simulink model "Project1_SPXMMA001"  (R2021a)
settings: Solver=ode1  StartTime=0.0  StopTime=Inf  RelTol=1e-3
InitFcn:
  |  TOFF_InitialValue.PRE = 12000;
  | OFF_InitialValue.PRE = 12000;
  | TON_InitialValue.PRE = 2000;
  | ON_InitialValue.PRE = 2000;
  | T2OFF_InitialValue.PRE = 11000;
  | T2ON_InitialValue.PRE = 3000;
  | T3OFF_InitialValue.PRE = 5000;
undefined symbols (not defined in the file): BOOL, DINT, slplc
libraries: simulink x7
(part 1 of 13)
settings Model: EnablePacing=on  Creator=arnoldpretorius  LastModifiedBy=Franc
settings SolverCC: AlgebraicLoopSolver=TrustRegion
settings DebuggingCC: SFMachineParentedDataDiag=warning

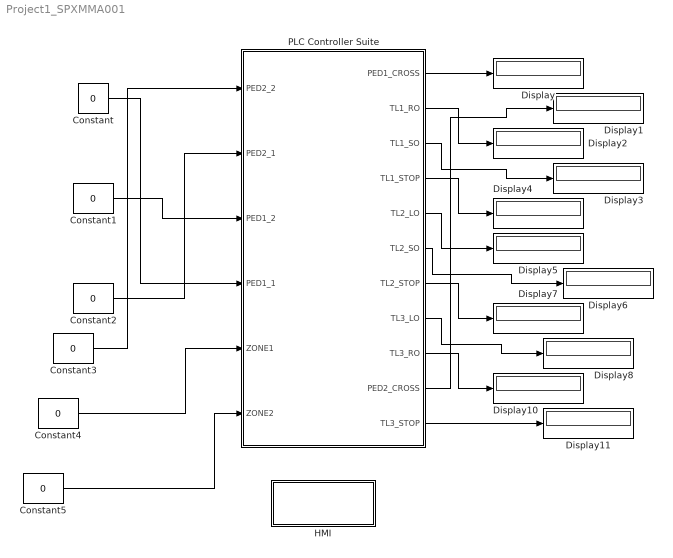
== system Project1_SPXMMA001 ==
  Constant{,1..5} (6 alike) : Constant  Value=0  OutDataTypeStr=boolean
  Display{,1..8,10..11} (11 alike) : Display
  HMI : Subsystem
  PLC Controller Suite : Subsystem  TreatAsAtomicUnit=on  mask{PLCBlockType=PLCController, PLCPOUType=PLC Controller}
      mask init:
      | slplc.callbacks.initController(gcb);
      settings: OpenFcn=slplc.callbacks.openPOUBlock(gcb);
      mask Help: web([docroot '/plccoder/ref/plccontrollersuite' '.html']);
      mask DialogControl PLCBlockTitle Prompt: PLC Controller Block
  wires:
  Constant/1 -> PLC Controller Suite/4(PED1_1)
  Constant1/1 -> PLC Controller Suite/3(PED1_2)
  Constant2/1 -> PLC Controller Suite/2(PED2_1)
  Constant3/1 -> PLC Controller Suite/1(PED2_2)
  PLC Controller Suite/1(PED1_CROSS) -> Display/1
  PLC Controller Suite/10(PED2_CROSS) -> Display1/1
  PLC Controller Suite/2(TL1_RO) -> Display2/1
  PLC Controller Suite/3(TL1_SO) -> Display3/1
  PLC Controller Suite/4(TL1_STOP) -> Display4/1
  PLC Controller Suite/5(TL2_LO) -> Display5/1
  PLC Controller Suite/6(TL2_SO) -> Display6/1
  PLC Controller Suite/7(TL2_STOP) -> Display7/1
  PLC Controller Suite/8(TL3_LO) -> Display8/1
  PLC Controller Suite/9(TL3_RO) -> Display10/1
  PLC Controller Suite/11(TL3_STOP) -> Display11/1
  Constant4/1 -> PLC Controller Suite/5(ZONE1)
  Constant5/1 -> PLC Controller Suite/6(ZONE2)

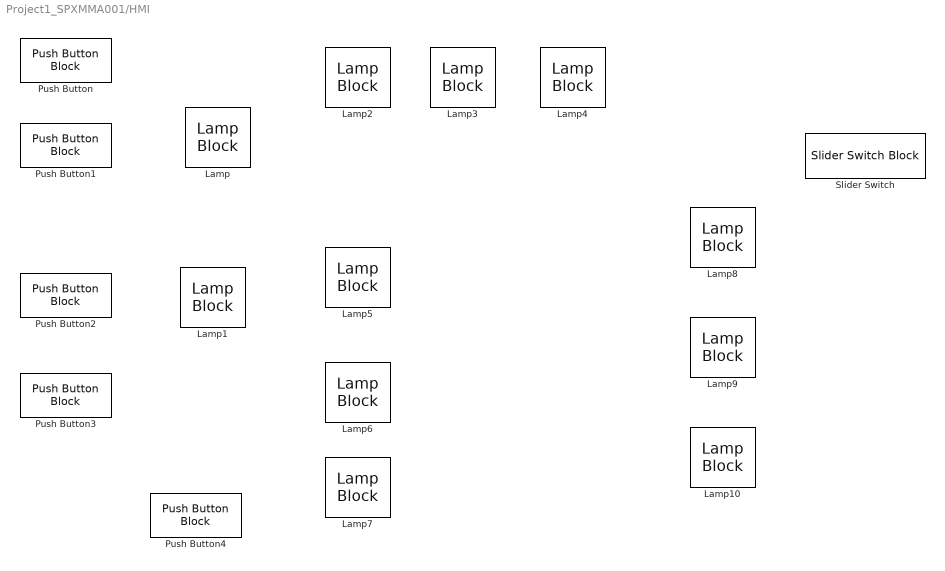
== system Project1_SPXMMA001/HMI ==
  Lamp{,1..10} (11 alike) : LampBlock
  Push Button : PushButtonBlock  ButtonText=PED1_1
  Push Button1 : PushButtonBlock  ButtonText=PED1_2
  Push Button2 : PushButtonBlock  ButtonText=PED2_1
  Push Button3 : PushButtonBlock  ButtonText=PED2_2
  Push Button4 : PushButtonBlock
  Slider Switch : SliderSwitchBlock  LabelPosition=Hide
      settings: Values={{'Off', 'On'}, [0 1]}

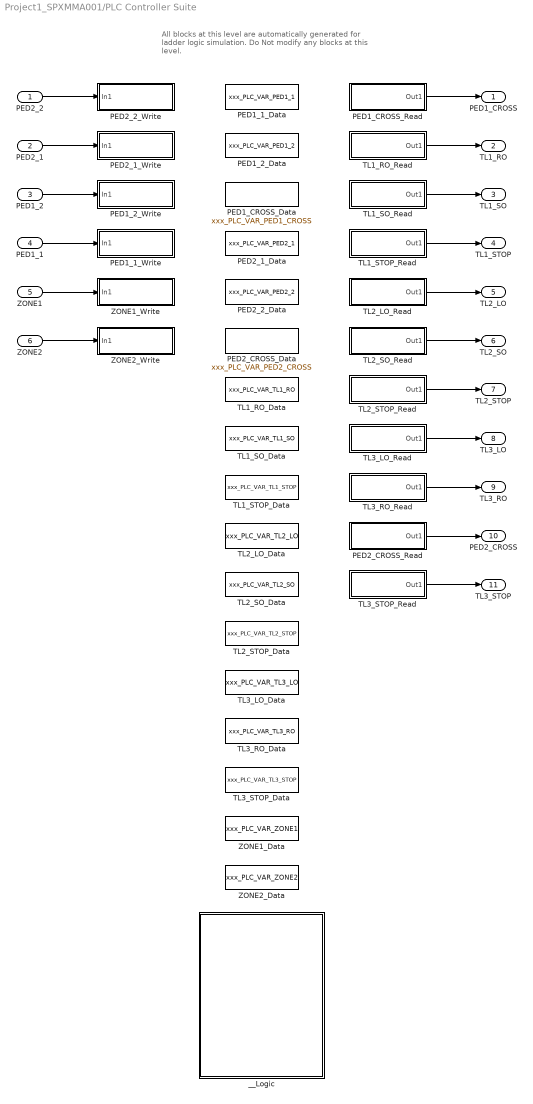
== system Project1_SPXMMA001/PLC Controller Suite ==
  note: All blocks at this level are automatically generated for ladder logic simulation.
      | Do Not modify any blocks at this level.
  PED2_2 : Inport  OutDataTypeStr=boolean
  PED2_1 : Inport  Port=2  OutDataTypeStr=boolean
  PED1_2 : Inport  Port=3  OutDataTypeStr=boolean
  PED1_1 : Inport  Port=4  OutDataTypeStr=boolean
  ZONE1 : Inport  Port=5  OutDataTypeStr=boolean
  ZONE2 : Inport  Port=6  OutDataTypeStr=boolean
  PED1_1_Data : DataStoreMemory  Tag=POUVariable  Priority=10  DataStoreName=xxx_PLC_VAR_PED1_1  ShowAdditionalParam=off  OutDataTypeStr=boolean  Dimensions=1
  PED1_1_Write : Subsystem  Priority=11  DisableCoverage=on  TreatAsAtomicUnit=on  mask{PLCOperandTag=PED1_1, PLCOperandExpression=xxx_PLC_VAR_PED1_1, PLCBlockType=VarWrite, PLCPOUType=VarWrite}
      mask prompts: PLCOperandTag "Operand Tag:"
      mask init:
      | slplc.callbacks.initInstruction(gcb);
      mask Help: web([docroot '/plccoder/ref/varwrite' '.html']);
      mask DialogControl PLCBlockTitle Prompt: Variable Write
      mask Display: disp(get_param(gcb, 'PLCOperandTag'));
  PED1_2_Data : DataStoreMemory  Tag=POUVariable  Priority=10  DataStoreName=xxx_PLC_VAR_PED1_2  ShowAdditionalParam=off  OutDataTypeStr=boolean  Dimensions=1
  PED1_2_Write : Subsystem  Priority=11  DisableCoverage=on  TreatAsAtomicUnit=on  mask{PLCOperandTag=PED1_2, PLCOperandExpression=xxx_PLC_VAR_PED1_2, PLCBlockType=VarWrite, PLCPOUType=VarWrite}
      mask prompts: PLCOperandTag "Operand Tag:"
      mask init:
      | slplc.callbacks.initInstruction(gcb);
      mask Help: web([docroot '/plccoder/ref/varwrite' '.html']);
      mask DialogControl PLCBlockTitle Prompt: Variable Write
      mask Display: disp(get_param(gcb, 'PLCOperandTag'));
  PED1_CROSS_Data : DataStoreMemory  Tag=POUVariable  Priority=10  DataStoreName=xxx_PLC_VAR_PED1_CROSS  ShowAdditionalParam=off  OutDataTypeStr=boolean  Dimensions=1
  PED1_CROSS_Read : Subsystem  Priority=13  DisableCoverage=on  TreatAsAtomicUnit=on  mask{PLCOperandTag=PED1_CROSS, PLCOperandExpression=xxx_PLC_VAR_PED1_CROSS, PLCBlockType=VarRead, PLCPOUType=VarRead}
      mask prompts: PLCOperandTag "Operand Tag"
      mask init:
      | block = gcb;
      | maskObj = Simulink.Mask.get(block);
      | maskObj.Display = sprintf('disp(''%s'');', PLCOperandTag);
      | slplc.callbacks.initInstruction(gcb);
      mask Help: web([docroot '/plccoder/ref/varread' '.html']);
      mask DialogControl PLCBlockTitle Prompt: Variable Read
      mask Display: disp('PED1_CROSS');
  PED2_1_Data : DataStoreMemory  Tag=POUVariable  Priority=10  DataStoreName=xxx_PLC_VAR_PED2_1  ShowAdditionalParam=off  OutDataTypeStr=boolean  Dimensions=1
  PED2_1_Write : Subsystem  Priority=11  DisableCoverage=on  TreatAsAtomicUnit=on  mask{PLCOperandTag=PED2_1, PLCOperandExpression=xxx_PLC_VAR_PED2_1, PLCBlockType=VarWrite, PLCPOUType=VarWrite}
      mask prompts: PLCOperandTag "Operand Tag:"
      mask init:
      | slplc.callbacks.initInstruction(gcb);
      mask Help: web([docroot '/plccoder/ref/varwrite' '.html']);
      mask DialogControl PLCBlockTitle Prompt: Variable Write
      mask Display: disp(get_param(gcb, 'PLCOperandTag'));
  PED2_2_Data : DataStoreMemory  Tag=POUVariable  Priority=10  DataStoreName=xxx_PLC_VAR_PED2_2  ShowAdditionalParam=off  OutDataTypeStr=boolean  Dimensions=1
  PED2_2_Write : Subsystem  Priority=11  DisableCoverage=on  TreatAsAtomicUnit=on  mask{PLCOperandTag=PED2_2, PLCOperandExpression=xxx_PLC_VAR_PED2_2, PLCBlockType=VarWrite, PLCPOUType=VarWrite}
      mask prompts: PLCOperandTag "Operand Tag:"
      mask init:
      | slplc.callbacks.initInstruction(gcb);
      mask Help: web([docroot '/plccoder/ref/varwrite' '.html']);
      mask DialogControl PLCBlockTitle Prompt: Variable Write
      mask Display: disp(get_param(gcb, 'PLCOperandTag'));
  PED2_CROSS_Data : DataStoreMemory  Tag=POUVariable  Priority=10  DataStoreName=xxx_PLC_VAR_PED2_CROSS  ShowAdditionalParam=off  OutDataTypeStr=boolean  Dimensions=1
  PED2_CROSS_Read : Subsystem  Priority=13  DisableCoverage=on  TreatAsAtomicUnit=on  mask{PLCOperandTag=PED2_CROSS, PLCOperandExpression=xxx_PLC_VAR_PED2_CROSS, PLCBlockType=VarRead, PLCPOUType=VarRead}
      mask prompts: PLCOperandTag "Operand Tag"
      mask init:
      | block = gcb;
      | maskObj = Simulink.Mask.get(block);
      | maskObj.Display = sprintf('disp(''%s'');', PLCOperandTag);
      | slplc.callbacks.initInstruction(gcb);
      mask Help: web([docroot '/plccoder/ref/varread' '.html']);
      mask DialogControl PLCBlockTitle Prompt: Variable Read
      mask Display: disp('PED2_CROSS');
  TL1_RO_Data : DataStoreMemory  Tag=POUVariable  Priority=10  DataStoreName=xxx_PLC_VAR_TL1_RO  ShowAdditionalParam=off  OutDataTypeStr=boolean  Dimensions=1
  TL1_RO_Read : Subsystem  Priority=13  DisableCoverage=on  TreatAsAtomicUnit=on  mask{PLCOperandTag=TL1_RO, PLCOperandExpression=xxx_PLC_VAR_TL1_RO, PLCBlockType=VarRead, PLCPOUType=VarRead}
      mask prompts: PLCOperandTag "Operand Tag"
      mask init:
      | block = gcb;
      | maskObj = Simulink.Mask.get(block);
      | maskObj.Display = sprintf('disp(''%s'');', PLCOperandTag);
      | slplc.callbacks.initInstruction(gcb);
      mask Help: web([docroot '/plccoder/ref/varread' '.html']);
      mask DialogControl PLCBlockTitle Prompt: Variable Read
      mask Display: disp('TL1_RO');
  TL1_SO_Data : DataStoreMemory  Tag=POUVariable  Priority=10  DataStoreName=xxx_PLC_VAR_TL1_SO  ShowAdditionalParam=off  OutDataTypeStr=boolean  Dimensions=1
  TL1_SO_Read : Subsystem  Priority=13  DisableCoverage=on  TreatAsAtomicUnit=on  mask{PLCOperandTag=TL1_SO, PLCOperandExpression=xxx_PLC_VAR_TL1_SO, PLCBlockType=VarRead, PLCPOUType=VarRead}
      mask prompts: PLCOperandTag "Operand Tag"
      mask init:
      | block = gcb;
      | maskObj = Simulink.Mask.get(block);
      | maskObj.Display = sprintf('disp(''%s'');', PLCOperandTag);
      | slplc.callbacks.initInstruction(gcb);
      mask Help: web([docroot '/plccoder/ref/varread' '.html']);
      mask DialogControl PLCBlockTitle Prompt: Variable Read
      mask Display: disp('TL1_SO');
  TL1_STOP_Data : DataStoreMemory  Tag=POUVariable  Priority=10  DataStoreName=xxx_PLC_VAR_TL1_STOP  ShowAdditionalParam=off  OutDataTypeStr=boolean  Dimensions=1
  TL1_STOP_Read : Subsystem  Priority=13  DisableCoverage=on  TreatAsAtomicUnit=on  mask{PLCOperandTag=TL1_STOP, PLCOperandExpression=xxx_PLC_VAR_TL1_STOP, PLCBlockType=VarRead, PLCPOUType=VarRead}
      mask prompts: PLCOperandTag "Operand Tag"
      mask init:
      | block = gcb;
      | maskObj = Simulink.Mask.get(block);
      | maskObj.Display = sprintf('disp(''%s'');', PLCOperandTag);
      | slplc.callbacks.initInstruction(gcb);
      mask Help: web([docroot '/plccoder/ref/varread' '.html']);
      mask DialogControl PLCBlockTitle Prompt: Variable Read
      mask Display: disp('TL1_STOP');
  TL2_LO_Data : DataStoreMemory  Tag=POUVariable  Priority=10  DataStoreName=xxx_PLC_VAR_TL2_LO  ShowAdditionalParam=off  OutDataTypeStr=boolean  Dimensions=1
  TL2_LO_Read : Subsystem  Priority=13  DisableCoverage=on  TreatAsAtomicUnit=on  mask{PLCOperandTag=TL2_LO, PLCOperandExpression=xxx_PLC_VAR_TL2_LO, PLCBlockType=VarRead, PLCPOUType=VarRead}
      mask prompts: PLCOperandTag "Operand Tag"
      mask init:
      | block = gcb;
      | maskObj = Simulink.Mask.get(block);
      | maskObj.Display = sprintf('disp(''%s'');', PLCOperandTag);
      | slplc.callbacks.initInstruction(gcb);
      mask Help: web([docroot '/plccoder/ref/varread' '.html']);
      mask DialogControl PLCBlockTitle Prompt: Variable Read
      mask Display: disp('TL2_LO');
  TL2_SO_Data : DataStoreMemory  Tag=POUVariable  Priority=10  DataStoreName=xxx_PLC_VAR_TL2_SO  ShowAdditionalParam=off  OutDataTypeStr=boolean  Dimensions=1
  TL2_SO_Read : Subsystem  Priority=13  DisableCoverage=on  TreatAsAtomicUnit=on  mask{PLCOperandTag=TL2_SO, PLCOperandExpression=xxx_PLC_VAR_TL2_SO, PLCBlockType=VarRead, PLCPOUType=VarRead}
      mask prompts: PLCOperandTag "Operand Tag"
      mask init:
      | block = gcb;
      | maskObj = Simulink.Mask.get(block);
      | maskObj.Display = sprintf('disp(''%s'');', PLCOperandTag);
      | slplc.callbacks.initInstruction(gcb);
      mask Help: web([docroot '/plccoder/ref/varread' '.html']);
      mask DialogControl PLCBlockTitle Prompt: Variable Read
      mask Display: disp('TL2_SO');
  TL2_STOP_Data : DataStoreMemory  Tag=POUVariable  Priority=10  DataStoreName=xxx_PLC_VAR_TL2_STOP  ShowAdditionalParam=off  OutDataTypeStr=boolean  Dimensions=1
  TL2_STOP_Read : Subsystem  Priority=13  DisableCoverage=on  TreatAsAtomicUnit=on  mask{PLCOperandTag=TL2_STOP, PLCOperandExpression=xxx_PLC_VAR_TL2_STOP, PLCBlockType=VarRead, PLCPOUType=VarRead}
      mask prompts: PLCOperandTag "Operand Tag"
      mask init:
      | block = gcb;
      | maskObj = Simulink.Mask.get(block);
      | maskObj.Display = sprintf('disp(''%s'');', PLCOperandTag);
      | slplc.callbacks.initInstruction(gcb);
      mask Help: web([docroot '/plccoder/ref/varread' '.html']);
      mask DialogControl PLCBlockTitle Prompt: Variable Read
      mask Display: disp('TL2_STOP');
  TL3_LO_Data : DataStoreMemory  Tag=POUVariable  Priority=10  DataStoreName=xxx_PLC_VAR_TL3_LO  ShowAdditionalParam=off  OutDataTypeStr=boolean  Dimensions=1
  TL3_LO_Read : Subsystem  Priority=13  DisableCoverage=on  TreatAsAtomicUnit=on  mask{PLCOperandTag=TL3_LO, PLCOperandExpression=xxx_PLC_VAR_TL3_LO, PLCBlockType=VarRead, PLCPOUType=VarRead}
      mask prompts: PLCOperandTag "Operand Tag"
      mask init:
      | block = gcb;
      | maskObj = Simulink.Mask.get(block);
      | maskObj.Display = sprintf('disp(''%s'');', PLCOperandTag);
      | slplc.callbacks.initInstruction(gcb);
      mask Help: web([docroot '/plccoder/ref/varread' '.html']);
      mask DialogControl PLCBlockTitle Prompt: Variable Read
      mask Display: disp('TL3_LO');
  TL3_RO_Data : DataStoreMemory  Tag=POUVariable  Priority=10  DataStoreName=xxx_PLC_VAR_TL3_RO  ShowAdditionalParam=off  OutDataTypeStr=boolean  Dimensions=1
  TL3_RO_Read : Subsystem  Priority=13  DisableCoverage=on  TreatAsAtomicUnit=on  mask{PLCOperandTag=TL3_RO, PLCOperandExpression=xxx_PLC_VAR_TL3_RO, PLCBlockType=VarRead, PLCPOUType=VarRead}
      mask prompts: PLCOperandTag "Operand Tag"
      mask init:
      | block = gcb;
      | maskObj = Simulink.Mask.get(block);
      | maskObj.Display = sprintf('disp(''%s'');', PLCOperandTag);
      | slplc.callbacks.initInstruction(gcb);
      mask Help: web([docroot '/plccoder/ref/varread' '.html']);
      mask DialogControl PLCBlockTitle Prompt: Variable Read
      mask Display: disp('TL3_RO');
  TL3_STOP_Data : DataStoreMemory  Tag=POUVariable  Priority=10  DataStoreName=xxx_PLC_VAR_TL3_STOP  ShowAdditionalParam=off  OutDataTypeStr=boolean  Dimensions=1
  TL3_STOP_Read : Subsystem  Priority=13  DisableCoverage=on  TreatAsAtomicUnit=on  mask{PLCOperandTag=TL3_STOP, PLCOperandExpression=xxx_PLC_VAR_TL3_STOP, PLCBlockType=VarRead, PLCPOUType=VarRead}
      mask prompts: PLCOperandTag "Operand Tag"
      mask init:
      | block = gcb;
      | maskObj = Simulink.Mask.get(block);
      | maskObj.Display = sprintf('disp(''%s'');', PLCOperandTag);
      | slplc.callbacks.initInstruction(gcb);
      mask Help: web([docroot '/plccoder/ref/varread' '.html']);
      mask DialogControl PLCBlockTitle Prompt: Variable Read
      mask Display: disp('TL3_STOP');
  ZONE1_Data : DataStoreMemory  Tag=POUVariable  Priority=10  DataStoreName=xxx_PLC_VAR_ZONE1  ShowAdditionalParam=off  OutDataTypeStr=boolean  Dimensions=1
  ZONE1_Write : Subsystem  Priority=11  DisableCoverage=on  TreatAsAtomicUnit=on  mask{PLCOperandTag=ZONE1, PLCOperandExpression=xxx_PLC_VAR_ZONE1, PLCBlockType=VarWrite, PLCPOUType=VarWrite}
      mask prompts: PLCOperandTag "Operand Tag:"
      mask init:
      | slplc.callbacks.initInstruction(gcb);
      mask Help: web([docroot '/plccoder/ref/varwrite' '.html']);
      mask DialogControl PLCBlockTitle Prompt: Variable Write
      mask Display: disp(get_param(gcb, 'PLCOperandTag'));
  ZONE2_Data : DataStoreMemory  Tag=POUVariable  Priority=10  DataStoreName=xxx_PLC_VAR_ZONE2  ShowAdditionalParam=off  OutDataTypeStr=boolean  Dimensions=1
  ZONE2_Write : Subsystem  Priority=11  DisableCoverage=on  TreatAsAtomicUnit=on  mask{PLCOperandTag=ZONE2, PLCOperandExpression=xxx_PLC_VAR_ZONE2, PLCBlockType=VarWrite, PLCPOUType=VarWrite}
      mask prompts: PLCOperandTag "Operand Tag:"
      mask init:
      | slplc.callbacks.initInstruction(gcb);
      mask Help: web([docroot '/plccoder/ref/varwrite' '.html']);
      mask DialogControl PLCBlockTitle Prompt: Variable Write
      mask Display: disp(get_param(gcb, 'PLCOperandTag'));
  __Logic : Subsystem  Priority=12  TreatAsAtomicUnit=on
  PED1_CROSS : Outport
  TL1_RO : Outport  Port=2
  TL1_SO : Outport  Port=3
  TL1_STOP : Outport  Port=4
  TL2_LO : Outport  Port=5
  TL2_SO : Outport  Port=6
  TL2_STOP : Outport  Port=7
  TL3_LO : Outport  Port=8
  TL3_RO : Outport  Port=9
  PED2_CROSS : Outport  Port=10
  TL3_STOP : Outport  Port=11
  wires:
  PED1_1/1 -> PED1_1_Write/1(In1)
  PED1_2/1 -> PED1_2_Write/1(In1)
  PED2_1/1 -> PED2_1_Write/1(In1)
  PED2_2/1 -> PED2_2_Write/1(In1)
  PED1_CROSS_Read/1(Out1) -> PED1_CROSS/1
  PED2_CROSS_Read/1(Out1) -> PED2_CROSS/1
  TL1_RO_Read/1(Out1) -> TL1_RO/1
  TL1_SO_Read/1(Out1) -> TL1_SO/1
  TL1_STOP_Read/1(Out1) -> TL1_STOP/1
  TL2_LO_Read/1(Out1) -> TL2_LO/1
  TL2_SO_Read/1(Out1) -> TL2_SO/1
  TL2_STOP_Read/1(Out1) -> TL2_STOP/1
  TL3_LO_Read/1(Out1) -> TL3_LO/1
  TL3_RO_Read/1(Out1) -> TL3_RO/1
  TL3_STOP_Read/1(Out1) -> TL3_STOP/1
  ZONE1/1 -> ZONE1_Write/1(In1)
  ZONE2/1 -> ZONE2_Write/1(In1)

== system Project1_SPXMMA001/PLC Controller Suite/PED1_1_Write ==
  In1 : Inport
  __CoreVarWrite : Subsystem  Tag=CoreVarWriteBlock  DisableCoverage=on  TreatAsAtomicUnit=on  mask{PLCBlockType=CoreVarWrite}
      mask init:
      | slplc.callbacks.initCoreVariable(gcb, 'write');
      mask DialogControl PLCBlockTitle Prompt: Core Variable Write
  wires:
  In1/1 -> __CoreVarWrite/1(u)

== system Project1_SPXMMA001/PLC Controller Suite/PED1_2_Write ==
  In1 : Inport
  __CoreVarWrite : Subsystem  Tag=CoreVarWriteBlock  DisableCoverage=on  TreatAsAtomicUnit=on  mask{PLCBlockType=CoreVarWrite}
      mask init:
      | slplc.callbacks.initCoreVariable(gcb, 'write');
      mask DialogControl PLCBlockTitle Prompt: Core Variable Write
  wires:
  In1/1 -> __CoreVarWrite/1(u)

== system Project1_SPXMMA001/PLC Controller Suite/PED1_CROSS_Read ==
  __CoreVarRead : Subsystem  Tag=CoreVarReadBlock  DisableCoverage=on  TreatAsAtomicUnit=on  mask{PLCBlockType=CoreVarRead}
      mask init:
      | slplc.callbacks.initCoreVariable(gcb, 'read');
      mask DialogControl PLCBlockTitle Prompt: Core Variable Read
  Out1 : Outport  VectorParamsAs1DForOutWhenUnconnected=off
  wires:
  __CoreVarRead/1(y) -> Out1/1

== system Project1_SPXMMA001/PLC Controller Suite/PED2_1_Write ==
  In1 : Inport
  __CoreVarWrite : Subsystem  Tag=CoreVarWriteBlock  DisableCoverage=on  TreatAsAtomicUnit=on  mask{PLCBlockType=CoreVarWrite}
      mask init:
      | slplc.callbacks.initCoreVariable(gcb, 'write');
      mask DialogControl PLCBlockTitle Prompt: Core Variable Write
  wires:
  In1/1 -> __CoreVarWrite/1(u)

== system Project1_SPXMMA001/PLC Controller Suite/PED2_2_Write ==
  In1 : Inport
  __CoreVarWrite : Subsystem  Tag=CoreVarWriteBlock  DisableCoverage=on  TreatAsAtomicUnit=on  mask{PLCBlockType=CoreVarWrite}
      mask init:
      | slplc.callbacks.initCoreVariable(gcb, 'write');
      mask DialogControl PLCBlockTitle Prompt: Core Variable Write
  wires:
  In1/1 -> __CoreVarWrite/1(u)

== system Project1_SPXMMA001/PLC Controller Suite/PED2_CROSS_Read ==
  __CoreVarRead : Subsystem  Tag=CoreVarReadBlock  DisableCoverage=on  TreatAsAtomicUnit=on  mask{PLCBlockType=CoreVarRead}
      mask init:
      | slplc.callbacks.initCoreVariable(gcb, 'read');
      mask DialogControl PLCBlockTitle Prompt: Core Variable Read
  Out1 : Outport  VectorParamsAs1DForOutWhenUnconnected=off
  wires:
  __CoreVarRead/1(y) -> Out1/1

== system Project1_SPXMMA001/PLC Controller Suite/TL1_RO_Read ==
  __CoreVarRead : Subsystem  Tag=CoreVarReadBlock  DisableCoverage=on  TreatAsAtomicUnit=on  mask{PLCBlockType=CoreVarRead}
      mask init:
      | slplc.callbacks.initCoreVariable(gcb, 'read');
      mask DialogControl PLCBlockTitle Prompt: Core Variable Read
  Out1 : Outport  VectorParamsAs1DForOutWhenUnconnected=off
  wires:
  __CoreVarRead/1(y) -> Out1/1

== system Project1_SPXMMA001/PLC Controller Suite/TL1_SO_Read ==
  __CoreVarRead : Subsystem  Tag=CoreVarReadBlock  DisableCoverage=on  TreatAsAtomicUnit=on  mask{PLCBlockType=CoreVarRead}
      mask init:
      | slplc.callbacks.initCoreVariable(gcb, 'read');
      mask DialogControl PLCBlockTitle Prompt: Core Variable Read
  Out1 : Outport  VectorParamsAs1DForOutWhenUnconnected=off
  wires:
  __CoreVarRead/1(y) -> Out1/1

== system Project1_SPXMMA001/PLC Controller Suite/TL1_STOP_Read ==
  __CoreVarRead : Subsystem  Tag=CoreVarReadBlock  DisableCoverage=on  TreatAsAtomicUnit=on  mask{PLCBlockType=CoreVarRead}
      mask init:
      | slplc.callbacks.initCoreVariable(gcb, 'read');
      mask DialogControl PLCBlockTitle Prompt: Core Variable Read
  Out1 : Outport  VectorParamsAs1DForOutWhenUnconnected=off
  wires:
  __CoreVarRead/1(y) -> Out1/1

== system Project1_SPXMMA001/PLC Controller Suite/TL2_LO_Read ==
  __CoreVarRead : Subsystem  Tag=CoreVarReadBlock  DisableCoverage=on  TreatAsAtomicUnit=on  mask{PLCBlockType=CoreVarRead}
      mask init:
      | slplc.callbacks.initCoreVariable(gcb, 'read');
      mask DialogControl PLCBlockTitle Prompt: Core Variable Read
  Out1 : Outport  VectorParamsAs1DForOutWhenUnconnected=off
  wires:
  __CoreVarRead/1(y) -> Out1/1

== system Project1_SPXMMA001/PLC Controller Suite/TL2_SO_Read ==
  __CoreVarRead : Subsystem  Tag=CoreVarReadBlock  DisableCoverage=on  TreatAsAtomicUnit=on  mask{PLCBlockType=CoreVarRead}
      mask init:
      | slplc.callbacks.initCoreVariable(gcb, 'read');
      mask DialogControl PLCBlockTitle Prompt: Core Variable Read
  Out1 : Outport  VectorParamsAs1DForOutWhenUnconnected=off
  wires:
  __CoreVarRead/1(y) -> Out1/1

== system Project1_SPXMMA001/PLC Controller Suite/TL2_STOP_Read ==
  __CoreVarRead : Subsystem  Tag=CoreVarReadBlock  DisableCoverage=on  TreatAsAtomicUnit=on  mask{PLCBlockType=CoreVarRead}
      mask init:
      | slplc.callbacks.initCoreVariable(gcb, 'read');
      mask DialogControl PLCBlockTitle Prompt: Core Variable Read
  Out1 : Outport  VectorParamsAs1DForOutWhenUnconnected=off
  wires:
  __CoreVarRead/1(y) -> Out1/1

== system Project1_SPXMMA001/PLC Controller Suite/TL3_LO_Read ==
  __CoreVarRead : Subsystem  Tag=CoreVarReadBlock  DisableCoverage=on  TreatAsAtomicUnit=on  mask{PLCBlockType=CoreVarRead}
      mask init:
      | slplc.callbacks.initCoreVariable(gcb, 'read');
      mask DialogControl PLCBlockTitle Prompt: Core Variable Read
  Out1 : Outport  VectorParamsAs1DForOutWhenUnconnected=off
  wires:
  __CoreVarRead/1(y) -> Out1/1

== system Project1_SPXMMA001/PLC Controller Suite/TL3_RO_Read ==
  __CoreVarRead : Subsystem  Tag=CoreVarReadBlock  DisableCoverage=on  TreatAsAtomicUnit=on  mask{PLCBlockType=CoreVarRead}
      mask init:
      | slplc.callbacks.initCoreVariable(gcb, 'read');
      mask DialogControl PLCBlockTitle Prompt: Core Variable Read
  Out1 : Outport  VectorParamsAs1DForOutWhenUnconnected=off
  wires:
  __CoreVarRead/1(y) -> Out1/1

== system Project1_SPXMMA001/PLC Controller Suite/TL3_STOP_Read ==
  __CoreVarRead : Subsystem  Tag=CoreVarReadBlock  DisableCoverage=on  TreatAsAtomicUnit=on  mask{PLCBlockType=CoreVarRead}
      mask init:
      | slplc.callbacks.initCoreVariable(gcb, 'read');
      mask DialogControl PLCBlockTitle Prompt: Core Variable Read
  Out1 : Outport  VectorParamsAs1DForOutWhenUnconnected=off
  wires:
  __CoreVarRead/1(y) -> Out1/1

== system Project1_SPXMMA001/PLC Controller Suite/ZONE1_Write ==
  In1 : Inport
  __CoreVarWrite : Subsystem  Tag=CoreVarWriteBlock  DisableCoverage=on  TreatAsAtomicUnit=on  mask{PLCBlockType=CoreVarWrite}
      mask init:
      | slplc.callbacks.initCoreVariable(gcb, 'write');
      mask DialogControl PLCBlockTitle Prompt: Core Variable Write
  wires:
  In1/1 -> __CoreVarWrite/1(u)

== system Project1_SPXMMA001/PLC Controller Suite/ZONE2_Write ==
  In1 : Inport
  __CoreVarWrite : Subsystem  Tag=CoreVarWriteBlock  DisableCoverage=on  TreatAsAtomicUnit=on  mask{PLCBlockType=CoreVarWrite}
      mask init:
      | slplc.callbacks.initCoreVariable(gcb, 'write');
      mask DialogControl PLCBlockTitle Prompt: Core Variable Write
  wires:
  In1/1 -> __CoreVarWrite/1(u)

== system Project1_SPXMMA001/PLC Controller Suite/__Logic ==
  Controller Tags : Subsystem  Tag=ControllerVariableSS  DisableCoverage=on  TreatAsAtomicUnit=on  mask{PLCVarPED2_2Name=PED2_2, PLCVarPED2_2Address=<empty>, PLCVarPED2_2Mapping=Input Symbol, PLCVarPED2_2PortIndex=1, PLCVarPED2_2DataType=boolean, PLCVarPED2_2Size=1, PLCVarPED2_2InitialValue=0, PLCVarPED2_2ToDelete=off, PLCVarPED2_1Name=PED2_1, PLCVarPED2_1Address=<empty>, PLCVarPED2_1Mapping=Input Symbol, PLCVarPED2_1PortIndex=2, PLCVarPED2_1DataType=boolean, PLCVarPED2_1Size=1, PLCVarPED2_1InitialValue=0, PLCVarPED2_1ToDelete=off, PLCVarPED1_2Name=PED1_2, PLCVarPED1_2Address=<empty>, PLCVarPED1_2Mapping=Input Symbol, PLCVarPED1_2PortIndex=3, PLCVarPED1_2DataType=boolean, PLCVarPED1_2Size=1, PLCVarPED1_2InitialValue=0, PLCVarPED1_2ToDelete=off, PLCVarPED1_1Name=PED1_1, PLCVarPED1_1Address=<empty>, PLCVarPED1_1Mapping=Input Symbol, PLCVarPED1_1PortIndex=4, PLCVarPED1_1DataType=boolean, PLCVarPED1_1Size=1, PLCVarPED1_1InitialValue=0, PLCVarPED1_1ToDelete=off, PLCVarZONE1Name=ZONE1, PLCVarZONE1Address=<empty>, PLCVarZONE1Mapping=Input Symbol, PLCVarZONE1PortIndex=5, PLCVarZONE1DataType=boolean, PLCVarZONE1Size=1, PLCVarZONE1InitialValue=0, PLCVarZONE1ToDelete=off, PLCVarZONE2Name=ZONE2, PLCVarZONE2Address=<empty>, PLCVarZONE2Mapping=Input Symbol, PLCVarZONE2PortIndex=6, PLCVarZONE2DataType=boolean, PLCVarZONE2Size=1, PLCVarZONE2InitialValue=0, PLCVarZONE2ToDelete=off, PLCVarPED1_CROSSName=PED1_CROSS, PLCVarPED1_CROSSAddress=<empty>, PLCVarPED1_CROSSMapping=Output Symbol, PLCVarPED1_CROSSPortIndex=1, PLCVarPED1_CROSSDataType=boolean, PLCVarPED1_CROSSSize=1, PLCVarPED1_CROSSInitialValue=0, PLCVarPED1_CROSSToDelete=off, PLCVarTL1_ROName=TL1_RO, PLCVarTL1_ROAddress=<empty>, PLCVarTL1_ROMapping=Output Symbol, PLCVarTL1_ROPortIndex=2, PLCVarTL1_RODataType=boolean, PLCVarTL1_ROSize=1, PLCVarTL1_ROInitialValue=0, PLCVarTL1_ROToDelete=off, PLCVarTL1_SOName=TL1_SO, PLCVarTL1_SOAddress=<empty>, PLCVarTL1_SOMapping=Output Symbol, PLCVarTL1_SOPortIndex=3, PLCVarTL1_SODataType=boolean, PLCVarTL1_SOSize=1, PLCVarTL1_SOInitialValue=0, PLCVarTL1_SOToDelete=off, PLCVarTL1_STOPName=TL1_STOP, PLCVarTL1_STOPAddress=<empty>, PLCVarTL1_STOPMapping=Output Symbol, PLCVarTL1_STOPPortIndex=4, PLCVarTL1_STOPDataType=boolean, PLCVarTL1_STOPSize=1, PLCVarTL1_STOPInitialValue=0, PLCVarTL1_STOPToDelete=off, PLCVarTL2_LOName=TL2_LO, PLCVarTL2_LOAddress=<empty>, PLCVarTL2_LOMapping=Output Symbol, PLCVarTL2_LOPortIndex=5, PLCVarTL2_LODataType=boolean, PLCVarTL2_LOSize=1, PLCVarTL2_LOInitialValue=0, PLCVarTL2_LOToDelete=off, PLCVarTL2_SOName=TL2_SO, PLCVarTL2_SOAddress=<empty>, PLCVarTL2_SOMapping=Output Symbol, PLCVarTL2_SOPortIndex=6, PLCVarTL2_SODataType=boolean, PLCVarTL2_SOSize=1, PLCVarTL2_SOInitialValue=0, PLCVarTL2_SOToDelete=off, PLCVarTL2_STOPName=TL2_STOP, PLCVarTL2_STOPAddress=<empty>, PLCVarTL2_STOPMapping=Output Symbol, PLCVarTL2_STOPPortIndex=7, PLCVarTL2_STOPDataType=boolean, PLCVarTL2_STOPSize=1, PLCVarTL2_STOPInitialValue=0, PLCVarTL2_STOPToDelete=off, PLCVarTL3_LOName=TL3_LO, PLCVarTL3_LOAddress=<empty>, PLCVarTL3_LOMapping=Output Symbol, PLCVarTL3_LOPortIndex=8, PLCVarTL3_LODataType=boolean, PLCVarTL3_LOSize=1, PLCVarTL3_LOInitialValue=0, PLCVarTL3_LOToDelete=off, PLCVarTL3_ROName=TL3_RO, PLCVarTL3_ROAddress=<empty>, PLCVarTL3_ROMapping=Output Symbol, PLCVarTL3_ROPortIndex=9, PLCVarTL3_RODataType=boolean, PLCVarTL3_ROSize=1, PLCVarTL3_ROInitialValue=0, PLCVarTL3_ROToDelete=off, PLCVarPED2_CROSSName=PED2_CROSS, PLCVarPED2_CROSSAddress=<empty>, PLCVarPED2_CROSSMapping=Output Symbol, PLCVarPED2_CROSSPortIndex=10, PLCVarPED2_CROSSDataType=boolean, PLCVarPED2_CROSSSize=1, PLCVarPED2_CROSSInitialValue=0, PLCVarPED2_CROSSToDelete=off, PLCVarTL3_STOPName=TL3_STOP, PLCVarTL3_STOPAddress=<empty>, PLCVarTL3_STOPMapping=Output Symbol, PLCVarTL3_STOPPortIndex=11, PLCVarTL3_STOPDataType=boolean, PLCVarTL3_STOPSize=1, PLCVarTL3_STOPInitialValue=0, PLCVarTL3_STOPToDelete=off}
      mask init:
      | slplc.callbacks.initControllerVarSS(gcb);
      settings: OpenFcn=slplc.callbacks.openControllerVariableSS(gcb);
      mask Help: web([docroot '/plccoder/ref/controllertags' '.html']);
      mask TypeOptions PLCVarPED2_2Mapping: Global Variable | Input Symbol | Output Symbol
      mask Callback PLCVarPED2_2Mapping: slplc.callbacks.updateControllerVarSS(gcb);
      mask TypeOptions PLCVarPED2_2PortIndex: 1 | 2 | 3 | 4 | 5 | 6 | 7 | 8 | 9 | 10 | 11 | 12 | 13 | 14 | 15 | 16 | 17
      mask TypeOptions PLCVarPED2_1Mapping: Global Variable | Input Symbol | Output Symbol
      mask Callback PLCVarPED2_1Mapping: slplc.callbacks.updateControllerVarSS(gcb);
      mask TypeOptions PLCVarPED2_1PortIndex: 1 | 2 | 3 | 4 | 5 | 6 | 7 | 8 | 9 | 10 | 11 | 12 | 13 | 14 | 15 | 16 | 17
      mask TypeOptions PLCVarPED1_2Mapping: Global Variable | Input Symbol | Output Symbol
      mask Callback PLCVarPED1_2Mapping: slplc.callbacks.updateControllerVarSS(gcb);
      mask TypeOptions PLCVarPED1_2PortIndex: 1 | 2 | 3 | 4 | 5 | 6 | 7 | 8 | 9 | 10 | 11 | 12 | 13 | 14 | 15 | 16 | 17
      mask TypeOptions PLCVarPED1_1Mapping: Global Variable | Input Symbol | Output Symbol
      mask Callback PLCVarPED1_1Mapping: slplc.callbacks.updateControllerVarSS(gcb);
      mask TypeOptions PLCVarPED1_1PortIndex: 1 | 2 | 3 | 4 | 5 | 6 | 7 | 8 | 9 | 10 | 11 | 12 | 13 | 14 | 15 | 16 | 17
      mask TypeOptions PLCVarZONE1Mapping: Global Variable | Input Symbol | Output Symbol
      mask Callback PLCVarZONE1Mapping: slplc.callbacks.updateControllerVarSS(gcb);
      mask TypeOptions PLCVarZONE1PortIndex: 1 | 2 | 3 | 4 | 5 | 6 | 7 | 8 | 9 | 10 | 11 | 12 | 13 | 14 | 15 | 16 | 17
      mask TypeOptions PLCVarZONE2Mapping: Global Variable | Input Symbol | Output Symbol
      mask Callback PLCVarZONE2Mapping: slplc.callbacks.updateControllerVarSS(gcb);
      mask TypeOptions PLCVarZONE2PortIndex: 1 | 2 | 3 | 4 | 5 | 6 | 7 | 8 | 9 | 10 | 11 | 12 | 13 | 14 | 15 | 16 | 17
      mask TypeOptions PLCVarPED1_CROSSMapping: Global Variable | Input Symbol | Output Symbol
      mask Callback PLCVarPED1_CROSSMapping: slplc.callbacks.updateControllerVarSS(gcb);
      mask TypeOptions PLCVarPED1_CROSSPortIndex: 1 | 2 | 3 | 4 | 5 | 6 | 7 | 8 | 9 | 10 | 11 | 12 | 13 | 14 | 15 | 16 | 17
      mask TypeOptions PLCVarTL1_ROMapping: Global Variable | Input Symbol | Output Symbol
      mask Callback PLCVarTL1_ROMapping: slplc.callbacks.updateControllerVarSS(gcb);
      mask TypeOptions PLCVarTL1_ROPortIndex: 1 | 2 | 3 | 4 | 5 | 6 | 7 | 8 | 9 | 10 | 11 | 12 | 13 | 14 | 15 | 16 | 17
      mask TypeOptions PLCVarTL1_SOMapping: Global Variable | Input Symbol | Output Symbol
      mask Callback PLCVarTL1_SOMapping: slplc.callbacks.updateControllerVarSS(gcb);
      mask TypeOptions PLCVarTL1_SOPortIndex: 1 | 2 | 3 | 4 | 5 | 6 | 7 | 8 | 9 | 10 | 11 | 12 | 13 | 14 | 15 | 16 | 17
      mask TypeOptions PLCVarTL1_STOPMapping: Global Variable | Input Symbol | Output Symbol
      mask Callback PLCVarTL1_STOPMapping: slplc.callbacks.updateControllerVarSS(gcb);
      mask TypeOptions PLCVarTL1_STOPPortIndex: 1 | 2 | 3 | 4 | 5 | 6 | 7 | 8 | 9 | 10 | 11 | 12 | 13 | 14 | 15 | 16 | 17
      mask TypeOptions PLCVarTL2_LOMapping: Global Variable | Input Symbol | Output Symbol
      mask Callback PLCVarTL2_LOMapping: slplc.callbacks.updateControllerVarSS(gcb);
      mask TypeOptions PLCVarTL2_LOPortIndex: 1 | 2 | 3 | 4 | 5 | 6 | 7 | 8 | 9 | 10 | 11 | 12 | 13 | 14 | 15 | 16 | 17
      mask TypeOptions PLCVarTL2_SOMapping: Global Variable | Input Symbol | Output Symbol
      mask Callback PLCVarTL2_SOMapping: slplc.callbacks.updateControllerVarSS(gcb);
      mask TypeOptions PLCVarTL2_SOPortIndex: 1 | 2 | 3 | 4 | 5 | 6 | 7 | 8 | 9 | 10 | 11 | 12 | 13 | 14 | 15 | 16 | 17
      mask TypeOptions PLCVarTL2_STOPMapping: Global Variable | Input Symbol | Output Symbol
      mask Callback PLCVarTL2_STOPMapping: slplc.callbacks.updateControllerVarSS(gcb);
      mask TypeOptions PLCVarTL2_STOPPortIndex: 1 | 2 | 3 | 4 | 5 | 6 | 7 | 8 | 9 | 10 | 11 | 12 | 13 | 14 | 15 | 16 | 17
      mask TypeOptions PLCVarTL3_LOMapping: Global Variable | Input Symbol | Output Symbol
      mask Callback PLCVarTL3_LOMapping: slplc.callbacks.updateControllerVarSS(gcb);
      mask TypeOptions PLCVarTL3_LOPortIndex: 1 | 2 | 3 | 4 | 5 | 6 | 7 | 8 | 9 | 10 | 11 | 12 | 13 | 14 | 15 | 16 | 17
      mask TypeOptions PLCVarTL3_ROMapping: Global Variable | Input Symbol | Output Symbol
      mask Callback PLCVarTL3_ROMapping: slplc.callbacks.updateControllerVarSS(gcb);
      mask TypeOptions PLCVarTL3_ROPortIndex: 1 | 2 | 3 | 4 | 5 | 6 | 7 | 8 | 9 | 10 | 11 | 12 | 13 | 14 | 15 | 16 | 17
      mask TypeOptions PLCVarPED2_CROSSMapping: Global Variable | Input Symbol | Output Symbol
      mask Callback PLCVarPED2_CROSSMapping: slplc.callbacks.updateControllerVarSS(gcb);
      mask TypeOptions PLCVarPED2_CROSSPortIndex: 1 | 2 | 3 | 4 | 5 | 6 | 7 | 8 | 9 | 10 | 11 | 12 | 13 | 14 | 15 | 16 | 17
      mask TypeOptions PLCVarTL3_STOPMapping: Global Variable | Input Symbol | Output Symbol
      mask Callback PLCVarTL3_STOPMapping: slplc.callbacks.updateControllerVarSS(gcb);
      mask TypeOptions PLCVarTL3_STOPPortIndex: 1 | 2 | 3 | 4 | 5 | 6 | 7 | 8 | 9 | 10 | 11 | 12 | 13 | 14 | 15 | 16 | 17
      mask DialogControl PLCBlockTitle Prompt: Global Variable and Symbol Spreadsheet
      mask DialogControl PLCVarListHeaderName Prompt: Name
      mask DialogControl PLCVarListHeaderAddress Prompt: Address (At)
      mask DialogControl PLCVarListHeaderMapping Prompt: Mapping Type
      mask DialogControl PLCVarListHeaderPortIndex Prompt: Port
      mask DialogControl PLCVarListHeaderDataType Prompt: Data Type
      mask DialogControl PLCVarListHeaderSize Prompt: Size
      mask DialogControl PLCVarListHeaderInitialValue Prompt: Initial Value
      mask DialogControl PLCVarListHeaderToDelete Prompt: Delete
  Task : Subsystem  TreatAsAtomicUnit=on  mask{PLCBlockType=Task, PLCPOUType=Task, PLCTaskWatchDog=0}
      settings: OpenFcn=slplc.callbacks.openTaskBlock(gcb);
      mask Help: web([docroot '/plccoder/ref/task' '.html']);
      mask DialogControl PLCBlockTitle Prompt: Task
  Up to Parent POU : Subsystem  DisableCoverage=on  TreatAsAtomicUnit=on  mask{PLCBlockType=OpenParentPOU}
      settings: OpenFcn=slplc.callbacks.openParentPOUBlock(gcb);
      mask Help: web([docroot '/plccoder/ref/uptoparentpou' '.html']);
      mask DialogControl PLCBlockTitle Prompt: Add Single Rung

== system Project1_SPXMMA001/PLC Controller Suite/PED1_1_Write/__CoreVarWrite ==
  u : Inport
  DataWrite : DataStoreWrite  DataStoreName=xxx_PLC_VAR_PED1_1  IndexOptions=Index vector (dialog)  Indices=1  OutputSizes=1
  wires:
  u/1 -> DataWrite/1

== system Project1_SPXMMA001/PLC Controller Suite/PED1_2_Write/__CoreVarWrite ==
  u : Inport
  DataWrite : DataStoreWrite  DataStoreName=xxx_PLC_VAR_PED1_2  IndexOptions=Index vector (dialog)  Indices=1  OutputSizes=1
  wires:
  u/1 -> DataWrite/1

== system Project1_SPXMMA001/PLC Controller Suite/PED1_CROSS_Read/__CoreVarRead ==
  DataRead : DataStoreRead  DataStoreName=xxx_PLC_VAR_PED1_CROSS  IndexOptions=Index vector (dialog)  Indices=1  OutputSizes=1
  y : Outport  VectorParamsAs1DForOutWhenUnconnected=off
  wires:
  DataRead/1 -> y/1

== system Project1_SPXMMA001/PLC Controller Suite/PED2_1_Write/__CoreVarWrite ==
  u : Inport
  DataWrite : DataStoreWrite  DataStoreName=xxx_PLC_VAR_PED2_1  IndexOptions=Index vector (dialog)  Indices=1  OutputSizes=1
  wires:
  u/1 -> DataWrite/1

== system Project1_SPXMMA001/PLC Controller Suite/PED2_2_Write/__CoreVarWrite ==
  u : Inport
  DataWrite : DataStoreWrite  DataStoreName=xxx_PLC_VAR_PED2_2  IndexOptions=Index vector (dialog)  Indices=1  OutputSizes=1
  wires:
  u/1 -> DataWrite/1

== system Project1_SPXMMA001/PLC Controller Suite/PED2_CROSS_Read/__CoreVarRead ==
  DataRead : DataStoreRead  DataStoreName=xxx_PLC_VAR_PED2_CROSS  IndexOptions=Index vector (dialog)  Indices=1  OutputSizes=1
  y : Outport  VectorParamsAs1DForOutWhenUnconnected=off
  wires:
  DataRead/1 -> y/1

== system Project1_SPXMMA001/PLC Controller Suite/TL1_RO_Read/__CoreVarRead ==
  DataRead : DataStoreRead  DataStoreName=xxx_PLC_VAR_TL1_RO  IndexOptions=Index vector (dialog)  Indices=1  OutputSizes=1
  y : Outport  VectorParamsAs1DForOutWhenUnconnected=off
  wires:
  DataRead/1 -> y/1

== system Project1_SPXMMA001/PLC Controller Suite/TL1_SO_Read/__CoreVarRead ==
  DataRead : DataStoreRead  DataStoreName=xxx_PLC_VAR_TL1_SO  IndexOptions=Index vector (dialog)  Indices=1  OutputSizes=1
  y : Outport  VectorParamsAs1DForOutWhenUnconnected=off
  wires:
  DataRead/1 -> y/1

== system Project1_SPXMMA001/PLC Controller Suite/TL1_STOP_Read/__CoreVarRead ==
  DataRead : DataStoreRead  DataStoreName=xxx_PLC_VAR_TL1_STOP  IndexOptions=Index vector (dialog)  Indices=1  OutputSizes=1
  y : Outport  VectorParamsAs1DForOutWhenUnconnected=off
  wires:
  DataRead/1 -> y/1

== system Project1_SPXMMA001/PLC Controller Suite/TL2_LO_Read/__CoreVarRead ==
  DataRead : DataStoreRead  DataStoreName=xxx_PLC_VAR_TL2_LO  IndexOptions=Index vector (dialog)  Indices=1  OutputSizes=1
  y : Outport  VectorParamsAs1DForOutWhenUnconnected=off
  wires:
  DataRead/1 -> y/1

== system Project1_SPXMMA001/PLC Controller Suite/TL2_SO_Read/__CoreVarRead ==
  DataRead : DataStoreRead  DataStoreName=xxx_PLC_VAR_TL2_SO  IndexOptions=Index vector (dialog)  Indices=1  OutputSizes=1
  y : Outport  VectorParamsAs1DForOutWhenUnconnected=off
  wires:
  DataRead/1 -> y/1

== system Project1_SPXMMA001/PLC Controller Suite/TL2_STOP_Read/__CoreVarRead ==
  DataRead : DataStoreRead  DataStoreName=xxx_PLC_VAR_TL2_STOP  IndexOptions=Index vector (dialog)  Indices=1  OutputSizes=1
  y : Outport  VectorParamsAs1DForOutWhenUnconnected=off
  wires:
  DataRead/1 -> y/1

== system Project1_SPXMMA001/PLC Controller Suite/TL3_LO_Read/__CoreVarRead ==
  DataRead : DataStoreRead  DataStoreName=xxx_PLC_VAR_TL3_LO  IndexOptions=Index vector (dialog)  Indices=1  OutputSizes=1
  y : Outport  VectorParamsAs1DForOutWhenUnconnected=off
  wires:
  DataRead/1 -> y/1

== system Project1_SPXMMA001/PLC Controller Suite/TL3_RO_Read/__CoreVarRead ==
  DataRead : DataStoreRead  DataStoreName=xxx_PLC_VAR_TL3_RO  IndexOptions=Index vector (dialog)  Indices=1  OutputSizes=1
  y : Outport  VectorParamsAs1DForOutWhenUnconnected=off
  wires:
  DataRead/1 -> y/1

== system Project1_SPXMMA001/PLC Controller Suite/TL3_STOP_Read/__CoreVarRead ==
  DataRead : DataStoreRead  DataStoreName=xxx_PLC_VAR_TL3_STOP  IndexOptions=Index vector (dialog)  Indices=1  OutputSizes=1
  y : Outport  VectorParamsAs1DForOutWhenUnconnected=off
  wires:
  DataRead/1 -> y/1

== system Project1_SPXMMA001/PLC Controller Suite/ZONE1_Write/__CoreVarWrite ==
  u : Inport
  DataWrite : DataStoreWrite  DataStoreName=xxx_PLC_VAR_ZONE1  IndexOptions=Index vector (dialog)  Indices=1  OutputSizes=1
  wires:
  u/1 -> DataWrite/1

== system Project1_SPXMMA001/PLC Controller Suite/ZONE2_Write/__CoreVarWrite ==
  u : Inport
  DataWrite : DataStoreWrite  DataStoreName=xxx_PLC_VAR_ZONE2  IndexOptions=Index vector (dialog)  Indices=1  OutputSizes=1
  wires:
  u/1 -> DataWrite/1

== system Project1_SPXMMA001/PLC Controller Suite/__Logic/Controller Tags ==

== system Project1_SPXMMA001/PLC Controller Suite/__Logic/Task ==
  Program : Subsystem  TreatAsAtomicUnit=on  mask{PLCPOUType=Program, PLCPOULanguage=LD, PLCBlockType=LDProgram}
      mask prompts: PLCPOUType "POU Type:"
      mask init:
      | slplc.callbacks.initProgram(gcb);
      settings: OpenFcn=slplc.callbacks.openPOUBlock(gcb);
      mask Help: web([docroot '/plccoder/ref/ldprogram' '.html']);
      mask DialogControl PLCBlockTitle Prompt: Program
      mask DialogControl PLCEditPOU Prompt: Edit POU
      mask DialogControl PLCEditInterface Prompt: Edit Variables
  Up to Parent POU : Subsystem  DisableCoverage=on  TreatAsAtomicUnit=on  mask{PLCBlockType=OpenParentPOU}
      settings: OpenFcn=slplc.callbacks.openParentPOUBlock(gcb);
      mask Help: web([docroot '/plccoder/ref/uptoparentpou' '.html']);
      mask DialogControl PLCBlockTitle Prompt: Add Single Rung

== system Project1_SPXMMA001/PLC Controller Suite/__Logic/Up to Parent POU ==

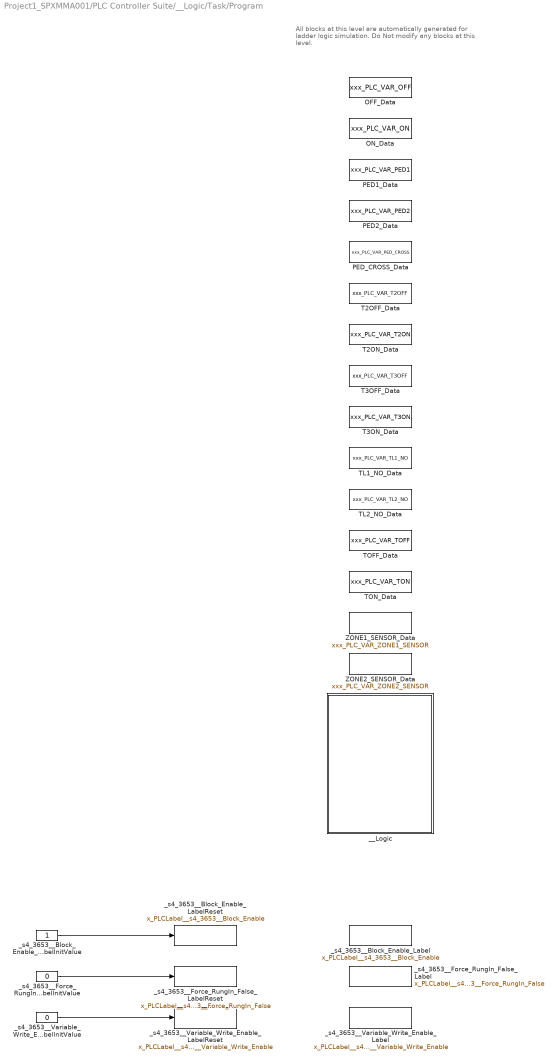
== system Project1_SPXMMA001/PLC Controller Suite/__Logic/Task/Program ==
  note: All blocks at this level are automatically generated for ladder logic simulation.
      | Do Not modify any blocks at this level.
  OFF_Data : DataStoreMemory  Tag=POUVariable  Priority=10  DataStoreName=xxx_PLC_VAR_OFF  InitialValue=OFF_InitialValue  ShowAdditionalParam=off  OutDataTypeStr=Bus: TIMER  Dimensions=1
  ON_Data : DataStoreMemory  Tag=POUVariable  Priority=10  DataStoreName=xxx_PLC_VAR_ON  InitialValue=ON_InitialValue  ShowAdditionalParam=off  OutDataTypeStr=Bus: TIMER  Dimensions=1
  PED1_Data : DataStoreMemory  Tag=POUVariable  Priority=10  DataStoreName=xxx_PLC_VAR_PED1  InitialValue=false  ShowAdditionalParam=off  OutDataTypeStr=BOOL  Dimensions=1
  PED2_Data : DataStoreMemory  Tag=POUVariable  Priority=10  DataStoreName=xxx_PLC_VAR_PED2  InitialValue=false  ShowAdditionalParam=off  OutDataTypeStr=boolean  Dimensions=1
  PED_CROSS_Data : DataStoreMemory  Tag=POUVariable  Priority=10  DataStoreName=xxx_PLC_VAR_PED_CROSS  InitialValue=false  ShowAdditionalParam=off  OutDataTypeStr=BOOL  Dimensions=1
  T2OFF_Data : DataStoreMemory  Tag=POUVariable  Priority=10  DataStoreName=xxx_PLC_VAR_T2OFF  InitialValue=T2OFF_InitialValue  ShowAdditionalParam=off  OutDataTypeStr=Bus: TIMER  Dimensions=1
  T2ON_Data : DataStoreMemory  Tag=POUVariable  Priority=10  DataStoreName=xxx_PLC_VAR_T2ON  InitialValue=T2ON_InitialValue  ShowAdditionalParam=off  OutDataTypeStr=Bus: TIMER  Dimensions=1
  T3OFF_Data : DataStoreMemory  Tag=POUVariable  Priority=10  DataStoreName=xxx_PLC_VAR_T3OFF  InitialValue=TOF_InitialValue  ShowAdditionalParam=off  OutDataTypeStr=Bus: TIMER  Dimensions=1
  T3ON_Data : DataStoreMemory  Tag=POUVariable  Priority=10  DataStoreName=xxx_PLC_VAR_T3ON  InitialValue=TON_InitialValue  ShowAdditionalParam=off  OutDataTypeStr=Bus: TIMER  Dimensions=1
  TL1_NO_Data : DataStoreMemory  Tag=POUVariable  Priority=10  DataStoreName=xxx_PLC_VAR_TL1_NO  InitialValue=false  ShowAdditionalParam=off  OutDataTypeStr=BOOL  Dimensions=1
  TL2_NO_Data : DataStoreMemory  Tag=POUVariable  Priority=10  DataStoreName=xxx_PLC_VAR_TL2_NO  InitialValue=false  ShowAdditionalParam=off  OutDataTypeStr=BOOL  Dimensions=1
  TOFF_Data : DataStoreMemory  Tag=POUVariable  Priority=10  DataStoreName=xxx_PLC_VAR_TOFF  InitialValue=TOFF_InitialValue  ShowAdditionalParam=off  OutDataTypeStr=Bus: TIMER  Dimensions=1
  TON_Data : DataStoreMemory  Tag=POUVariable  Priority=10  DataStoreName=xxx_PLC_VAR_TON  InitialValue=TON_InitialValue  ShowAdditionalParam=off  OutDataTypeStr=Bus: TIMER  Dimensions=1
  ZONE1_SENSOR_Data : DataStoreMemory  Tag=POUVariable  Priority=10  DataStoreName=xxx_PLC_VAR_ZONE1_SENSOR  InitialValue=false  ShowAdditionalParam=off  OutDataTypeStr=BOOL  Dimensions=1
  ZONE2_SENSOR_Data : DataStoreMemory  Tag=POUVariable  Priority=10  DataStoreName=xxx_PLC_VAR_ZONE2_SENSOR  InitialValue=false  ShowAdditionalParam=off  OutDataTypeStr=BOOL  Dimensions=1
  __Logic : Subsystem  Priority=12  TreatAsAtomicUnit=on
  _s4_3653__Block_Enable_Label : DataStoreMemory  Priority=10  DataStoreName=x_PLCLabel__s4_3653__Block_Enable  InitialValue=1  ShowAdditionalParam=off  OutDataTypeStr=BOOL  Dimensions=1
  _s4_3653__Block_Enable_LabelInitValue : Constant  OutDataTypeStr=BOOL
  _s4_3653__Block_Enable_LabelReset : DataStoreWrite  Priority=11  DataStoreName=x_PLCLabel__s4_3653__Block_Enable  IndexOptions=Index vector (dialog)  Indices=1  OutputSizes=1
  _s4_3653__Force_RungIn_False_Label : DataStoreMemory  Priority=10  DataStoreName=x_PLCLabel__s4_3653__Force_RungIn_False  ShowAdditionalParam=off  OutDataTypeStr=BOOL  Dimensions=1
  _s4_3653__Force_RungIn_False_LabelInitValue : Constant  Value=0  OutDataTypeStr=BOOL
  _s4_3653__Force_RungIn_False_LabelReset : DataStoreWrite  Priority=11  DataStoreName=x_PLCLabel__s4_3653__Force_RungIn_False  IndexOptions=Index vector (dialog)  Indices=1  OutputSizes=1
  _s4_3653__Variable_Write_Enable_Label : DataStoreMemory  Priority=10  DataStoreName=x_PLCLabel__s4_3653__Variable_Write_Enable  ShowAdditionalParam=off  OutDataTypeStr=BOOL  Dimensions=1
  _s4_3653__Variable_Write_Enable_LabelInitValue : Constant  Value=0  OutDataTypeStr=BOOL
  _s4_3653__Variable_Write_Enable_LabelReset : DataStoreWrite  Priority=11  DataStoreName=x_PLCLabel__s4_3653__Variable_Write_Enable  IndexOptions=Index vector (dialog)  Indices=1  OutputSizes=1
  wires:
  _s4_3653__Block_Enable_LabelInitValue/1 -> _s4_3653__Block_Enable_LabelReset/1
  _s4_3653__Variable_Write_Enable_LabelInitValue/1 -> _s4_3653__Variable_Write_Enable_LabelReset/1
  _s4_3653__Force_RungIn_False_LabelInitValue/1 -> _s4_3653__Force_RungIn_False_LabelReset/1

== system Project1_SPXMMA001/PLC Controller Suite/__Logic/Task/Up to Parent POU ==
